simulink model "CRA_Assignment7_linearized"  (R2022b)
settings: Solver=VariableStepAuto  StartTime=0.0  StopTime=5.5  RelTol=1e-9  AbsTol=1e-5
settings Model: Creator=Andrea  LastModifiedBy=Andrea

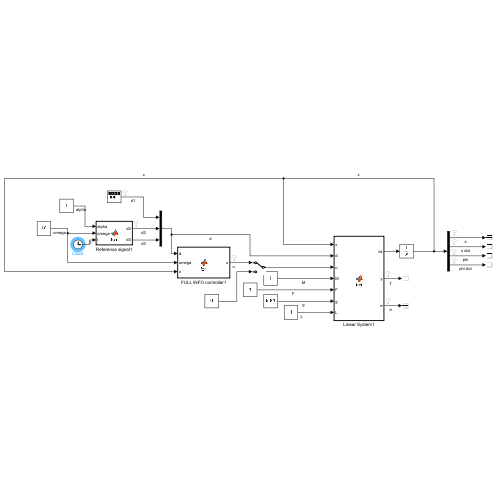
[thumbnail: Simulink's stored preview of the top-level diagram]
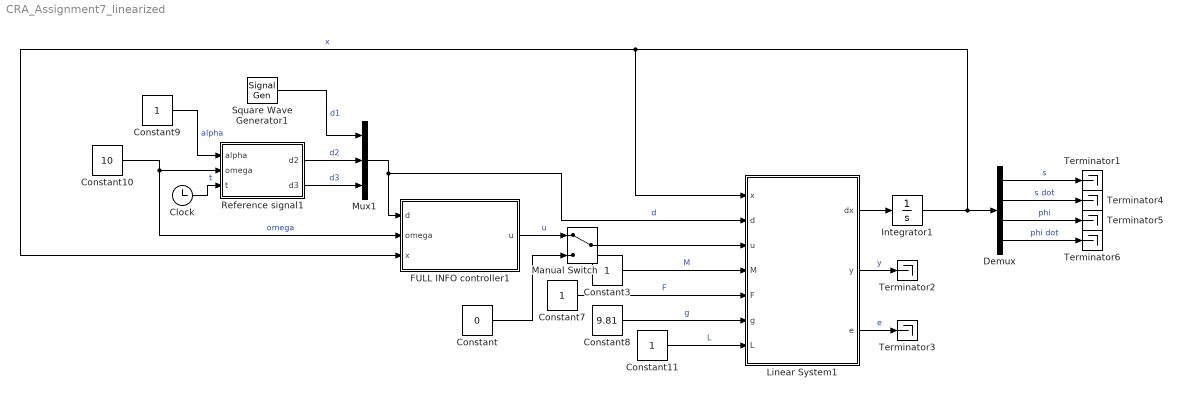
== system CRA_Assignment7_linearized ==
  Clock : Clock
  Constant : Constant  Value=0
  Constant10 : Constant  Value=10
  Constant{3,7,9,11} (4 alike) : Constant
  Constant8 : Constant  Value=9.81
  Demux : Demux
  FULL INFO controller1 : MATLAB Function  TreatAsAtomicUnit=on
  Integrator1 : Integrator  InitialCondition=[0,0,0,0]  ContinuousStateAttributes='position_and_angle'
  Linear System1 : MATLAB Function  TreatAsAtomicUnit=on
  Manual Switch : ManualSwitch
  Mux1 : Mux  Inputs=3
  Reference signal1 : MATLAB Function  TreatAsAtomicUnit=on
  Square Wave Generator1 : SignalGenerator  WaveForm=square  Amplitude=0.5  Frequency=0.02*2*3.16  Units=rad/sec
  Terminator{1..6} (6 alike) : Terminator
  wires:
  Constant11/1 -> Linear System1/7(L)  "L"
  Constant10/1 -> FULL INFO controller1/2(omega), Reference signal1/2(omega)  "omega"
  Square Wave Generator1/1 -> Mux1/1  "d1"
  Clock/1 -> Reference signal1/3(t)  "t"
  Integrator1/1 -> FULL INFO controller1/3(x), Linear System1/1(x), Demux/1  "x"
  Constant9/1 -> Reference signal1/1(alpha)  "alpha"
  Linear System1/1(dx) -> Integrator1/1
  Reference signal1/1(d2) -> Mux1/2  "d2"
  Mux1/1 -> FULL INFO controller1/1(d), Linear System1/2(d)  "d"
  Reference signal1/2(d3) -> Mux1/3  "d3"
  Constant8/1 -> Linear System1/6(g)  "g"
  Linear System1/3(e) -> Terminator3/1  "e"
  Constant3/1 -> Linear System1/4(M)  "M"
  Linear System1/2(y) -> Terminator2/1  "y"
  Constant7/1 -> Linear System1/5(F)  "F"
  Demux/1 -> Terminator1/1  "s"
  Demux/2 -> Terminator4/1  "s dot"
  Demux/3 -> Terminator5/1  "phi"
  Demux/4 -> Terminator6/1  "phi dot"
  FULL INFO controller1/1(u) -> Manual Switch/1  "u"
  Manual Switch/1 -> Linear System1/3(u)
  Constant/1 -> Manual Switch/2

== matlab function CRA_Assignment7_linearized/FULL INFO controller1 ==
  data: d input; omega input; u output; x input
function u = fcn(d,omega,x)
% FULL INFO CONTROLLER  u=K*x+(Γ-K*Π)*d

Kx = 15.09683995922528*x(4)+47.25648318042813*x(3)+6.09683995922528*x(2)+2.446483180428134*x(1);
Ld = d(3)*((15.09683995922528*omega^3)/(omega^2+9.81)-5.09683995922528*omega)+d(2)*((47.25648318042813*omega^2)/(omega^2+9.81)-omega^2-2.446483180428134)-1.0*d(1);
u = Kx + Ld;

== matlab function CRA_Assignment7_linearized/Linear System1 ==
  data: x input; d input; dx output; u input; y output; M input; F input; g input; e output; L input
function [dx,y,e] = fcn(x,d,u,M,F,g,L)
A = [0,    1,   0,  0;
     0, -F/M,   0,  0;
     0,    0,   0,  1;
     0, F/(L*M), g/L,  0];
 
B = [    0;
       1/M;
         0;
     -1/(L*M)];

P = [   0, 0, 0;
      1/M, 0, 0;
        0, 0, 0;
    -1/(L*M), 0, 0];

dx = (A*x + B*u + P*d)';


y = [x(2), x(4)]';

e = d(2)-x(1);
end

== matlab function CRA_Assignment7_linearized/Reference signal1 ==
  data: alpha input; omega input; d2 output; t input; d3 output
function [d2,d3] = fcn(alpha,omega,t)
%#FULL INFO CONTROLLER  u=K*x+(Γ-K*Π)*d

d2 = alpha * sin(omega*t);
d3 = alpha * cos(omega*t);
end
